simulink model "Actuador"  (R2021a)
settings: Solver=VariableStepAuto  StartTime=0.0  StopTime=0.3  RelTol=1e-3
settings Model: Creator=luisd  LastModifiedBy=luisd

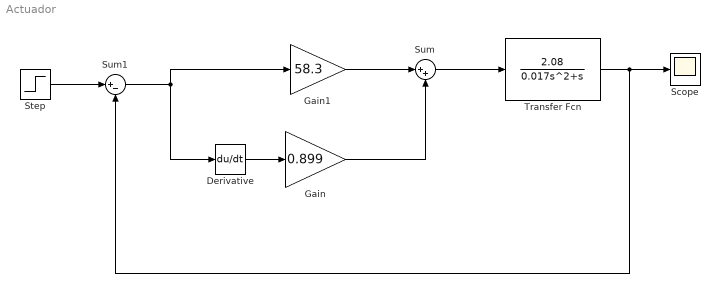
== system Actuador ==
  Derivative : Derivative
  Gain : Gain  Gain=0.899
  Gain1 : Gain  Gain=58.3
  Scope : Scope
  Step : Step  Time=0  After=12  SampleTime=0
  Sum : Sum  Inputs=|++
  Sum1 : Sum  Inputs=|+-
  Transfer Fcn : TransferFcn  Numerator=[2.08]  Denominator=[0.017 1 0]
  wires:
  Transfer Fcn/1 -> Sum1/2, Scope/1
  Sum/1 -> Transfer Fcn/1
  Gain/1 -> Sum/2
  Gain1/1 -> Sum/1
  Derivative/1 -> Gain/1
  Step/1 -> Sum1/1
  Sum1/1 -> Gain1/1, Derivative/1
